simulink model "model8"  (R2024b)
settings: Solver=VariableStepAuto  StartTime=0.0  StopTime=10.0  RelTol=1e-3
settings Model: Creator=kacpe  LastModifiedBy=kacpe

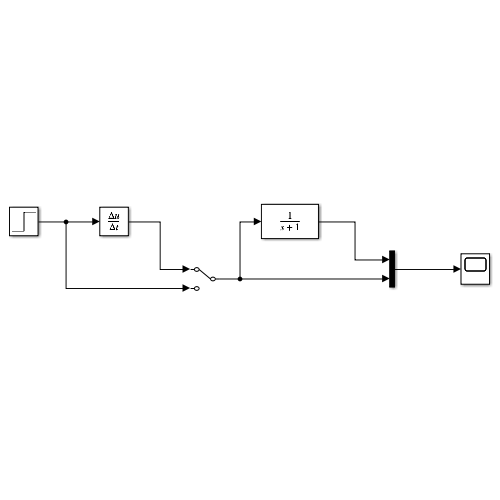
[thumbnail: Simulink's stored preview of the top-level diagram]
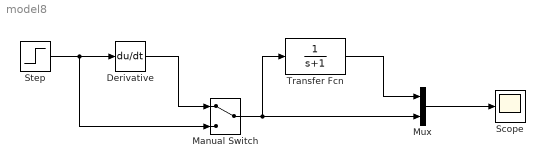
== system model8 ==
  Derivative : Derivative
  Manual Switch : ManualSwitch
  Mux : Mux  Inputs=2
  Scope : Scope
  Step : Step  SampleTime=0
  Transfer Fcn : TransferFcn  Denominator=[1 1]
  wires:
  Step/1 -> Manual Switch/2, Derivative/1
  Transfer Fcn/1 -> Mux/1
  Mux/1 -> Scope/1
  Manual Switch/1 -> Transfer Fcn/1, Mux/2
  Derivative/1 -> Manual Switch/1
